simulink model "untitled"  (R2017a)
settings: Solver=ode45  StartTime=0.0  StopTime=10  RelTol=1e-3
values from neighbouring files (symbols this model uses):
  Kd = 2    [pid_parameters.m]
  Ki = 10    [pid_parameters.m]
  Kp = 10    [pid_parameters.m]
libraries: nesl_utility x2, simulink x1, sm_lib x1
settings Model: Creator=Yogesh  LastModifiedBy=Yogesh

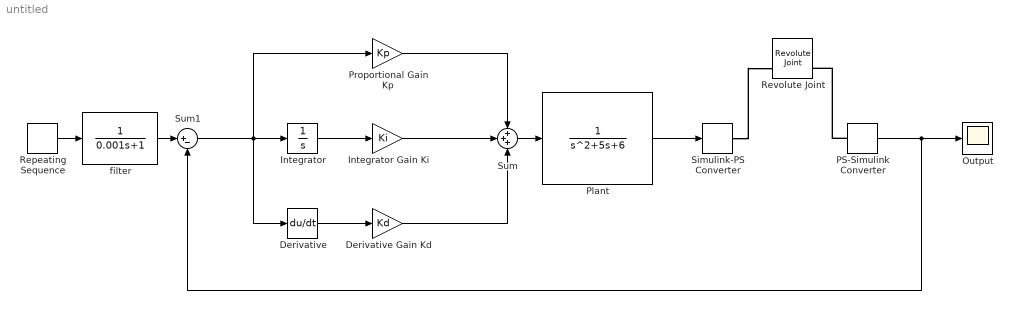
== system untitled ==
  Derivative : Derivative
  Derivative Gain Kd : Gain  Gain=Kd
  Integrator : Integrator
  Integrator Gain Ki : Gain  Gain=Ki
  Output : Scope
  PS-Simulink Converter : nesl_utility/PS-Simulink Converter  PhysicalDomain=network_engine_domain  SubClassName=ps_output  LeftPortType=input  RightPortType=output  PseudoPeriodic=off  Frequencies=[]  Unit=1  AffineConversion=off
  Plant : TransferFcn  Denominator=[1 5 6]
  Proportional Gain Kp : Gain  Gain=Kp
  Repeating Sequence : simulink/Sources/Repeating Sequence  rep_seq_t=time  rep_seq_y=signal
  Revolute Joint : sm_lib/Joints/Revolute Joint  SenseConstraintForce=off  SenseConstraintForceX=off  SenseConstraintForceY=off  SenseConstraintForceZ=off  SenseConstraintTorque=off  SenseConstraintTorqueX=off  SenseConstraintTorqueY=off  SenseConstraintTorqueZ=off  SenseTotalForce=off  SenseTotalForceX=off  SenseTotalForceY=off  SenseTotalForceZ=off  SenseTotalTorque=off  SenseTotalTorqueX=off  SenseTotalTorqueY=off  SenseTotalTorqueZ=off  CompositeWrenchDir=FollowerOnBase  CompositeWrenchFrame=BaseFrame  EquilibriumPosition=0  EquilibriumPositionUnits=deg  SpringStiffness=0  SpringStiffnessUnits=N*m/deg  DampingCoefficient=0  DampingCoefficientUnits=N*m/(deg/s)  TorqueActuationMode=NoTorque  MotionActuationMode=InputMotion  SensePosition=on  SenseVelocity=off  SenseAcceleration=off  SenseTorqueForce=off  PositionTargetSpecify=off  PositionTargetPriority=High  PositionTargetValue=0  PositionTargetValueUnits=deg  VelocityTargetSpecify=off  VelocityTargetPriority=High  VelocityTargetValue=0  VelocityTargetValueUnits=deg/s
  Simulink-PS Converter : nesl_utility/Simulink-PS Converter  PhysicalDomain=network_engine_domain  SubClassName=ps_input  LeftPortType=input  RightPortType=output  PseudoPeriodic=off  Frequencies=[]  NoiseDistribution=none  NoiseParameters=[]  Unit=deg  AffineConversion=off  FilteringAndDerivatives=filter  SimscapeFilterOrder=2  InputFilterTimeConstant=0.001  UdotUserProvided=0
  Sum : Sum  Inputs=3
  Sum1 : Sum  Inputs=|+-
  filter : TransferFcn  Denominator=[0.001 1]
  wires:
  Proportional Gain Kp/1 -> Sum/1
  Integrator/1 -> Integrator Gain Ki/1
  Derivative/1 -> Derivative Gain Kd/1
  Sum/1 -> Plant/1
  Sum1/1 -> Derivative/1, Integrator/1, Proportional Gain Kp/1
  Repeating Sequence/1 -> filter/1
  filter/1 -> Sum1/1
  Integrator Gain Ki/1 -> Sum/2
  Derivative Gain Kd/1 -> Sum/3
  PS-Simulink Converter/1 -> Sum1/2, Output/1
  Plant/1 -> Simulink-PS Converter/1
  connections:
  Simulink-PS Converter/RConn1 -- Revolute Joint/LConn2
  PS-Simulink Converter/LConn1 -- Revolute Joint/RConn2
